simulink model "configuring_inputs"  (R2023b)
settings: Solver=VariableStepAuto  StartTime=0.0  StopTime=10.0  RelTol=1e-3
settings Model: Creator=aryam  LastModifiedBy=aryam

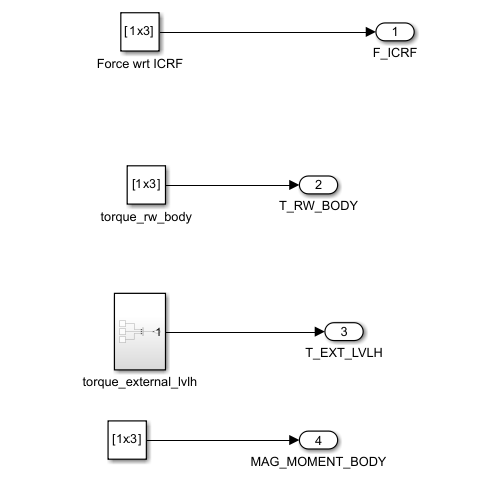
[thumbnail: Simulink's stored preview of the top-level diagram]
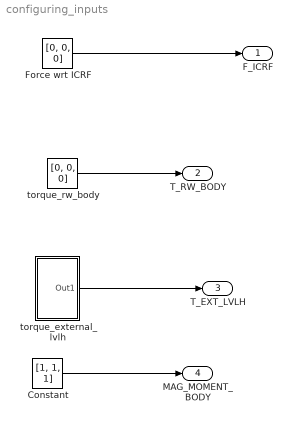
== system configuring_inputs ==
  Constant : Constant  Value=[1, 1, 1]
  Force wrt ICRF : Constant  Value="[0,  0, 0]"
  torque_external_lvlh : Subsystem
  torque_rw_body : Constant  Value=[0, 0, 0]
  F_ICRF : Outport
  T_RW_BODY : Outport  Port=2
  T_EXT_LVLH : Outport  Port=3
  "MAG_MOMENT_BODY " : Outport  Port=4
  wires:
  Force wrt ICRF/1 -> F_ICRF/1
  torque_rw_body/1 -> T_RW_BODY/1
  torque_external_lvlh/1(Out1) -> T_EXT_LVLH/1
  Constant/1 -> "MAG_MOMENT_BODY "/1

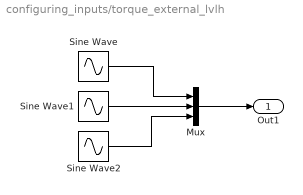
== system configuring_inputs/torque_external_lvlh ==
  Mux : Mux  Inputs=3
  Sine Wave : Sin  SampleTime=0
  Sine Wave1 : Sin  SampleTime=0
  Sine Wave2 : Sin  SampleTime=0
  Out1 : Outport
  wires:
  Sine Wave/1 -> Mux/1
  Sine Wave1/1 -> Mux/2
  Sine Wave2/1 -> Mux/3
  Mux/1 -> Out1/1
